simulink model "TD_1doF"  (R2019b)
settings: Solver=VariableStepAuto  StartTime=0.0  StopTime=50  RelTol=1e-3
undefined symbols (not defined in the file): Dm, Dt, g, Jp, k_pitch, Mb, w_neg, w_pos
settings Model: Creator=peter  LastModifiedBy=lbend

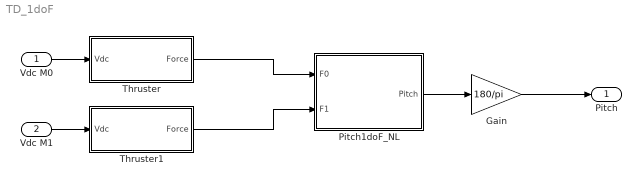
== system TD_1doF ==
  Vdc M0 : Inport
  Vdc M1 : Inport  Port=2
  Gain : Gain  Gain=180/pi
  Pitch1doF_NL : Subsystem
  Thruster : Subsystem
  Thruster1 : Subsystem
  Pitch : Outport
  wires:
  Thruster/1(Force) -> Pitch1doF_NL/1(F0)
  Thruster1/1(Force) -> Pitch1doF_NL/2("F1 ")
  Vdc M0/1 -> Thruster/1(Vdc)
  Pitch1doF_NL/1(Pitch) -> Gain/1
  Gain/1 -> Pitch/1
  Vdc M1/1 -> Thruster1/1(Vdc)

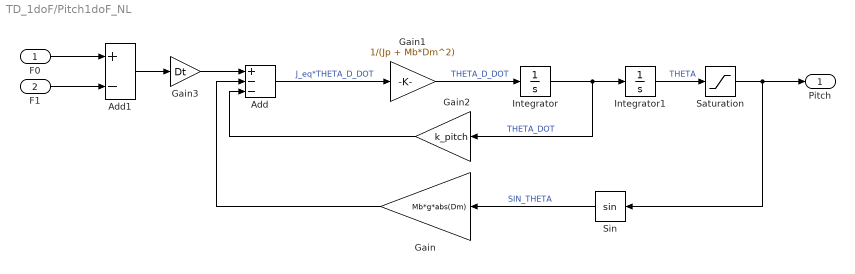
== system TD_1doF/Pitch1doF_NL ==
  F0 : Inport
  "F1 " : Inport  Port=2
  Add : Sum  Inputs=+--
  Add1 : Sum  Inputs=+-
  Gain : Gain  Gain=Mb*g*abs(Dm)
  Gain1 : Gain  Gain=1/(Jp + Mb*Dm^2)
  Gain2 : Gain  Gain=k_pitch
  Gain3 : Gain  Gain=Dt
  Integrator : Integrator
  Integrator1 : Integrator
  Saturation : Saturate  UpperLimit=0.93  LowerLimit=-0.93
  Sin : Trigonometry
  Pitch : Outport
  wires:
  Gain2/1 -> Add/3
  Saturation/1 -> Sin/1, Pitch/1
  Sin/1 -> Gain/1  "SIN_THETA"
  Integrator/1 -> Gain2/1, Integrator1/1  "THETA_DOT"
  Add/1 -> Gain1/1  "J_eq*THETA_D_DOT"
  Add1/1 -> Gain3/1
  Gain1/1 -> Integrator/1  "THETA_D_DOT"
  Gain3/1 -> Add/1
  Gain/1 -> Add/2
  "F1 "/1 -> Add1/2
  Integrator1/1 -> Saturation/1  "THETA"
  F0/1 -> Add1/1

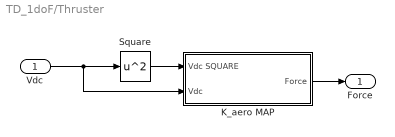
== system TD_1doF/Thruster ==
  Vdc : Inport
  K_aero MAP : Subsystem
  Square : Math  Operator=square  SignedPower=off  SaturateOnIntegerOverflow=on
  Force : Outport
  wires:
  Vdc/1 -> K_aero MAP/2(Vdc), Square/1
  Square/1 -> K_aero MAP/1(Vdc SQUARE)
  K_aero MAP/1(Force) -> Force/1

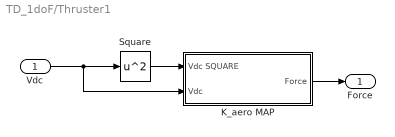
== system TD_1doF/Thruster1 ==
  Vdc : Inport
  K_aero MAP : Subsystem
  Square : Math  Operator=square  SignedPower=off  SaturateOnIntegerOverflow=on
  Force : Outport
  wires:
  Vdc/1 -> K_aero MAP/2(Vdc), Square/1
  Square/1 -> K_aero MAP/1(Vdc SQUARE)
  K_aero MAP/1(Force) -> Force/1

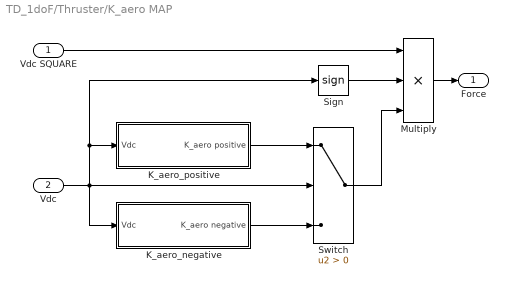
== system TD_1doF/Thruster/K_aero MAP ==
  Vdc SQUARE : Inport
  Vdc : Inport  Port=2
  K_aero_negative : Subsystem
  K_aero_positive : Subsystem
  "Multiply " : Product  Inputs=***
  Sign : Signum
  Switch : Switch  Criteria=u2 > Threshold
  Force : Outport
  wires:
  Vdc SQUARE/1 -> "Multiply "/1
  "Multiply "/1 -> Force/1
  Vdc/1 -> K_aero_negative/1(Vdc), Switch/2, Sign/1, K_aero_positive/1(Vdc)
  K_aero_positive/1(K_aero positive) -> Switch/1
  K_aero_negative/1(K_aero negative) -> Switch/3
  Switch/1 -> "Multiply "/3
  Sign/1 -> "Multiply "/2

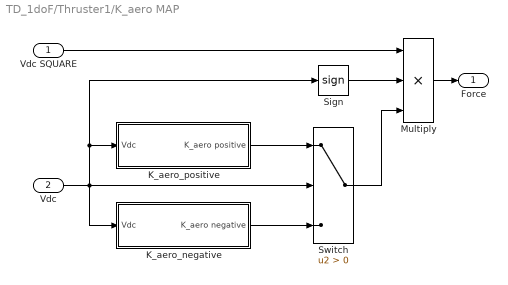
== system TD_1doF/Thruster1/K_aero MAP ==
  Vdc SQUARE : Inport
  Vdc : Inport  Port=2
  K_aero_negative : Subsystem
  K_aero_positive : Subsystem
  "Multiply " : Product  Inputs=***
  Sign : Signum
  Switch : Switch  Criteria=u2 > Threshold
  Force : Outport
  wires:
  Vdc SQUARE/1 -> "Multiply "/1
  "Multiply "/1 -> Force/1
  Vdc/1 -> K_aero_negative/1(Vdc), Switch/2, Sign/1, K_aero_positive/1(Vdc)
  K_aero_positive/1(K_aero positive) -> Switch/1
  K_aero_negative/1(K_aero negative) -> Switch/3
  Switch/1 -> "Multiply "/3
  Sign/1 -> "Multiply "/2

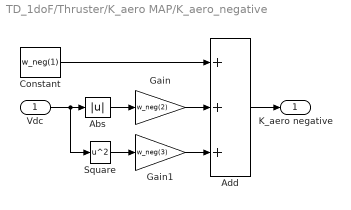
== system TD_1doF/Thruster/K_aero MAP/K_aero_negative ==
  Vdc : Inport
  Abs : Abs
  Add : Sum  Inputs=+++
  Constant : Constant  Value=w_neg(1)  SampleTime=0
  Gain : Gain  Gain=w_neg(2)
  Gain1 : Gain  Gain=w_neg(3)
  Square : Math  Operator=square  SignedPower=off  SaturateOnIntegerOverflow=on
  K_aero negative : Outport
  wires:
  Gain1/1 -> Add/3
  Add/1 -> K_aero negative/1
  Constant/1 -> Add/1
  Gain/1 -> Add/2
  Square/1 -> Gain1/1
  Abs/1 -> Gain/1
  Vdc/1 -> Square/1, Abs/1

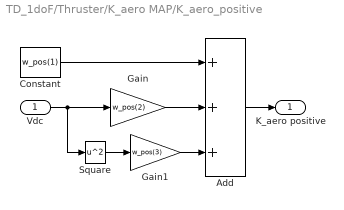
== system TD_1doF/Thruster/K_aero MAP/K_aero_positive ==
  Vdc : Inport
  Add : Sum  Inputs=+++
  Constant : Constant  Value=w_pos(1)  SampleTime=0
  Gain : Gain  Gain=w_pos(2)
  Gain1 : Gain  Gain=w_pos(3)
  Square : Math  Operator=square  SignedPower=off  SaturateOnIntegerOverflow=on
  K_aero positive : Outport
  wires:
  Constant/1 -> Add/1
  Vdc/1 -> Square/1, Gain/1
  Add/1 -> K_aero positive/1
  Gain/1 -> Add/2
  Square/1 -> Gain1/1
  Gain1/1 -> Add/3

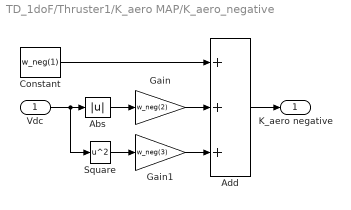
== system TD_1doF/Thruster1/K_aero MAP/K_aero_negative ==
  Vdc : Inport
  Abs : Abs
  Add : Sum  Inputs=+++
  Constant : Constant  Value=w_neg(1)  SampleTime=0
  Gain : Gain  Gain=w_neg(2)
  Gain1 : Gain  Gain=w_neg(3)
  Square : Math  Operator=square  SignedPower=off  SaturateOnIntegerOverflow=on
  K_aero negative : Outport
  wires:
  Gain1/1 -> Add/3
  Add/1 -> K_aero negative/1
  Constant/1 -> Add/1
  Gain/1 -> Add/2
  Square/1 -> Gain1/1
  Abs/1 -> Gain/1
  Vdc/1 -> Square/1, Abs/1

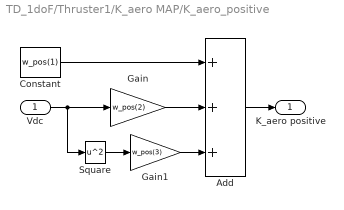
== system TD_1doF/Thruster1/K_aero MAP/K_aero_positive ==
  Vdc : Inport
  Add : Sum  Inputs=+++
  Constant : Constant  Value=w_pos(1)  SampleTime=0
  Gain : Gain  Gain=w_pos(2)
  Gain1 : Gain  Gain=w_pos(3)
  Square : Math  Operator=square  SignedPower=off  SaturateOnIntegerOverflow=on
  K_aero positive : Outport
  wires:
  Constant/1 -> Add/1
  Vdc/1 -> Square/1, Gain/1
  Add/1 -> K_aero positive/1
  Gain/1 -> Add/2
  Square/1 -> Gain1/1
  Gain1/1 -> Add/3
